simulink model "new_model"  (R2022b)
settings: Solver=VariableStepAuto  StartTime=0.0  StopTime=230  RelTol=1e-3
values from neighbouring files (symbols this model uses):
  stepAmplitude = 1    [idnet.m]
settings Model: Creator=DFUNDO  LastModifiedBy=DFUNDO

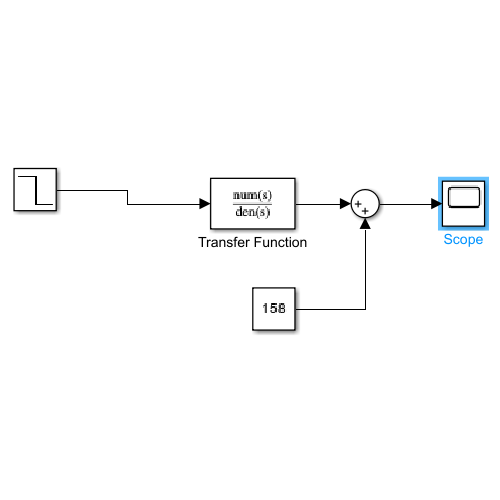
[thumbnail: Simulink's stored preview of the top-level diagram]
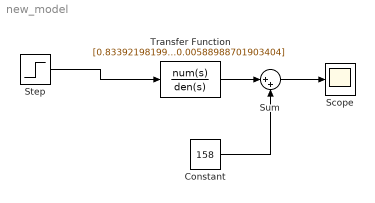
== system new_model ==
  Constant : Constant  Value=158
  Scope : Scope
  Step : Step  Before=stepAmplitude  After=0  SampleTime=0
  Sum : Sum  Inputs=|++
  Transfer Function : TransferFcn  Numerator=[0.833921981998895 -0.00140401381954936]  Denominator=[1 0.0940734789798433 0.00588988701903404]
  wires:
  Step/1 -> Transfer Function/1
  Sum/1 -> Scope/1
  Transfer Function/1 -> Sum/1
  Constant/1 -> Sum/2
